simulink model "TO_ctr"  (R2017b)
settings: Solver=ode4  StartTime=0.0  StopTime=10  FixedStep=0.001  RelTol=1e-3
undefined symbols (not defined in the file or in its folder): MPC_alfa_tracking, MPC_TO_des_trq, sigbuilder_block
settings Model: Creator=Yutong Li  LastModifiedBy=Yutong Li

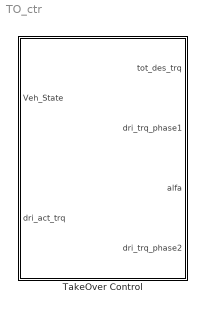
== system TO_ctr ==
  TakeOver Control : Subsystem

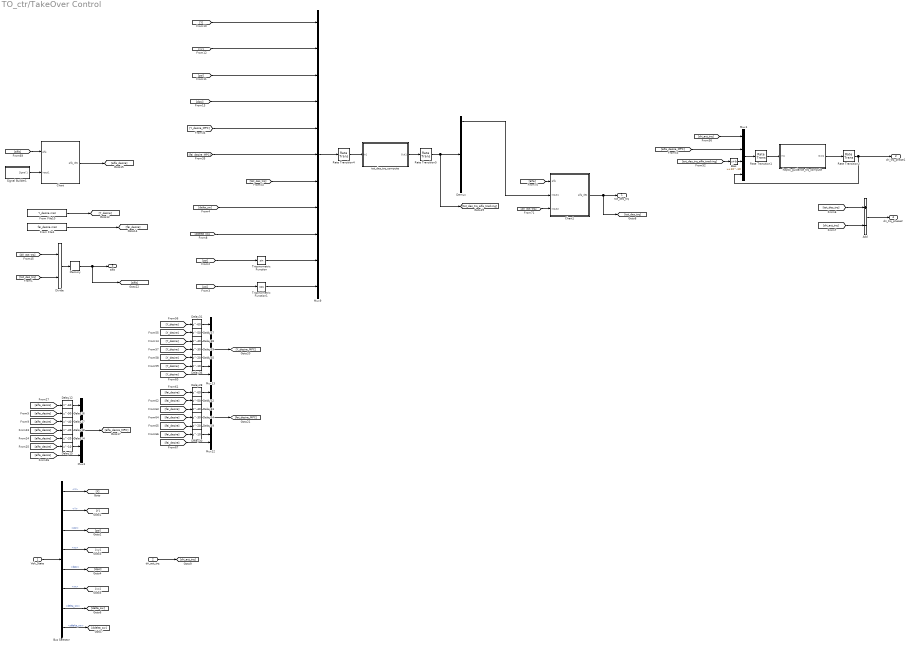
== system TO_ctr/TakeOver Control ==
  Veh_State : Inport
  dri_act_trq : Inport  Port=2
  Add : Sum  Inputs=+-
  Bias : Bias  Bias=10^-10
  Bus Selector : BusSelector  OutputSignals=X,Y,psi,vy,dpsi,vx,delta_sw,ddelta_sw
  Chart : Stateflow chart  TreatAsAtomicUnit=on
  Chart1 : Stateflow chart  TreatAsAtomicUnit=on
  Delay12 : Delay  DelayLength=60  InitialCondition=0
  Delay14 : Delay  DelayLength=20  InitialCondition=0
  Delay15 : Delay  DelayLength=10  InitialCondition=0
  Delay16 : Delay  DelayLength=50  InitialCondition=0
  Delay17 : Delay  DelayLength=40  InitialCondition=0
  Delay18 : Delay  DelayLength=30  InitialCondition=0
  Delay28 : Delay  DelayLength=60  InitialCondition=0
  Delay29 : Delay  DelayLength=20  InitialCondition=0
  Delay30 : Delay  DelayLength=10  InitialCondition=0
  Delay31 : Delay  DelayLength=60  InitialCondition=0
  Delay32 : Delay  DelayLength=50  InitialCondition=0
  Delay33 : Delay  DelayLength=40  InitialCondition=0
  Delay34 : Delay  DelayLength=30  InitialCondition=0
  Delay35 : Delay  DelayLength=20  InitialCondition=0
  Delay36 : Delay  DelayLength=10  InitialCondition=0
  Delay37 : Delay  DelayLength=50  InitialCondition=0
  Delay38 : Delay  DelayLength=40  InitialCondition=0
  Delay39 : Delay  DelayLength=30  InitialCondition=0
  Demux : Demux  Outputs=7
  Divide : Product  Inputs=*/
  From File1 : FromFile  FileName=fai_desire.mat
  From File10 : FromFile  FileName=Y_desire.mat
  Memory : Memory
  Mux1 : Mux
  Mux12 : Mux  Inputs=7
  Mux13 : Mux  Inputs=7
  Mux3 : Mux  Inputs=7
  Mux9 : Mux  Inputs=11
  Rate Transition1 : RateTransition  OutPortSampleTime=0.01
  Rate Transition2 : RateTransition
  Rate Transition4 : RateTransition  OutPortSampleTime=0.01
  Rate Transition5 : RateTransition
  Signal Builder1 : Subsystem  Tag=STV Subsys  LoadFcn=sigbuilder_block('load');  StartFcn=sigbuilder_block('start');  StopFcn=sigbuilder_block('stop');  ClipboardFcn=sigbuilder_block('clipboard');  mask(Sigbuilder block){tuvar=[0:10]}
      mask help: Simulink:masks:SigbuilderBlock_MD
      mask init:
      | if ~strcmp(get_param(bdroot(gcbh),'SimulationStatus'),'stopped') tuvar = sigbuilder_block('maskInit'); end
      settings: CopyFcn=sigbuilder_block('copy');  DeleteFcn=sigbuilder_block('delete');  ModelCloseFcn=sigbuilder_block('modelClose');  PreSaveFcn=sigbuilder_block('preSave');  PauseFcn=sigbuilder_block('pause');  ContinueFcn=sigbuilder_block('continue');  NameChangeFcn=sigbuilder_block('namechange');  OpenFcn=sigbuilder_block('open',[5.5 30 949 419 ]);  CloseFcn=sigbuilder_block('close');
      mask Display: plot(0, 0, 100, 100,[2, 2, 32, 32, 2], [68, 8, 8, 68, 68],[32, 2], [38, 38], [32, 19, 2],[53, 60, 44], [32, 17, 17, 2],[16, 16, 31, 31]);txt = getActiveGroup(gcbh);text(2, 100, txt,'verticalAlignment', 'top');
  Trigonometric Function : Trigonometry
  Trigonometric Function1 : Trigonometry  Operator=cos
  haptic_guidance_trq_compute : Subsystem  TreatAsAtomicUnit=on
  tot_des_trq_compute : Subsystem  TreatAsAtomicUnit=on
  tot_des_trq : Outport
  dri_trq_phase1 : Outport  Port=2
  alfa : Outport  Port=3
  dri_trq_phase2 : Outport  Port=4
  wires:
  Veh_State/1 -> Bus Selector/1
  Bus Selector/1 -> [X]  "<X>"
  Bus Selector/2 -> [Y]  "<Y>"
  Bus Selector/3 -> [psi]  "<psi>"
  Bus Selector/4 -> [vy]  "<vy>"
  Bus Selector/5 -> [dpsi]  "<dpsi>"
  Bus Selector/6 -> [vx]  "<vx>"
  [Y] -> Mux9/1
  [vy] -> Mux9/2
  [psi] -> Mux9/3
  [dpsi] -> Mux9/4
  From File10/1 -> [Y_desire]
  [alfa_desire] -> Delay14/1
  Delay16/1 -> Mux3/2
  [alfa_desire] -> Delay12/1
  [alfa_desire] -> Delay15/1
  [alfa_desire] -> Mux3/7
  [alfa_desire] -> Delay17/1
  Delay12/1 -> Mux3/1
  Delay14/1 -> Mux3/5
  Delay17/1 -> Mux3/3
  Delay18/1 -> Mux3/4
  [alfa_desire] -> Delay18/1
  [alfa_desire] -> Delay16/1
  Delay15/1 -> Mux3/6
  Mux3/1 -> [alfa_desire_MPC]
  [dri_act_trq] -> Divide/1
  [fai_desire_MPC] -> Mux9/6
  [Y_desire_MPC] -> Mux9/5
  Rate Transition4/1 -> tot_des_trq_compute/1(In1)
  tot_des_trq_compute/1(Out1) -> Rate Transition5/1
  Mux9/1 -> Rate Transition4/1
  Bus Selector/7 -> [delta_sw]  "<delta_sw>"
  Bus Selector/8 -> [ddelta_sw]  "<ddelta_sw>"
  [delta_sw] -> Mux9/8
  [ddelta_sw] -> Mux9/9
  [psi] -> Trigonometric Function/1
  Trigonometric Function/1 -> Mux9/10
  [psi] -> Trigonometric Function1/1
  Trigonometric Function1/1 -> Mux9/11
  Mux1/1 -> Rate Transition1/1
  Rate Transition1/1 -> haptic_guidance_trq_compute/1(In1)
  haptic_guidance_trq_compute/1(Out1) -> Rate Transition2/1
  Rate Transition2/1 -> dri_trq_phase1/1, Mux1/4
  dri_act_trq/1 -> [dri_act_trq]
  [tot_des_trq] -> Divide/2
  [dri_act_trq] -> Mux1/1
  [alfa_desire_MPC] -> Mux1/2
  [tot_des_trq_alfa_tracking] -> Bias/1
  Bias/1 -> Mux1/3
  Demux/1 -> Chart1/2(input1)
  [tot_des_trq] -> Mux9/7
  Rate Transition5/1 -> [tot_des_trq_alfa_tracking], Demux/1
  Mux12/1 -> [fai_desire_MPC]
  Delay36/1 -> Mux13/6
  Mux13/1 -> [Y_desire_MPC]
  [fai_desire] -> Delay29/1
  [fai_desire] -> Delay30/1
  [fai_desire] -> Delay33/1
  Delay29/1 -> Mux12/5
  Delay33/1 -> Mux12/3
  [fai_desire] -> Delay32/1
  Delay34/1 -> Mux12/4
  [Y_desire] -> Mux13/7
  [Y_desire] -> Delay38/1
  Delay37/1 -> Mux13/2
  [fai_desire] -> Delay28/1
  [Y_desire] -> Delay35/1
  Delay30/1 -> Mux12/6
  Delay38/1 -> Mux13/3
  [Y_desire] -> Delay37/1
  Delay32/1 -> Mux12/2
  [Y_desire] -> Delay39/1
  [fai_desire] -> Delay34/1
  [fai_desire] -> Mux12/7
  Delay31/1 -> Mux13/1
  Delay35/1 -> Mux13/5
  [Y_desire] -> Delay36/1
  Delay39/1 -> Mux13/4
  [Y_desire] -> Delay31/1
  Delay28/1 -> Mux12/1
  From File1/1 -> [fai_desire]
  Divide/1 -> Memory/1
  Signal Builder1/1(Signal 1) -> Chart/2(input1)
  Memory/1 -> [alfa], alfa/1
  Chart/1(alfa_des) -> [alfa_desire]
  [alfa] -> Chart/1(alfa)
  [alfa] -> Chart1/1(alfa)
  [dri_act_trq] -> Chart1/3(input2)
  Chart1/1(alfa_des) -> [tot_des_trq], tot_des_trq/1
  Add/1 -> dri_trq_phase2/1
  [tot_des_trq] -> Add/1
  [dri_act_trq] -> Add/2

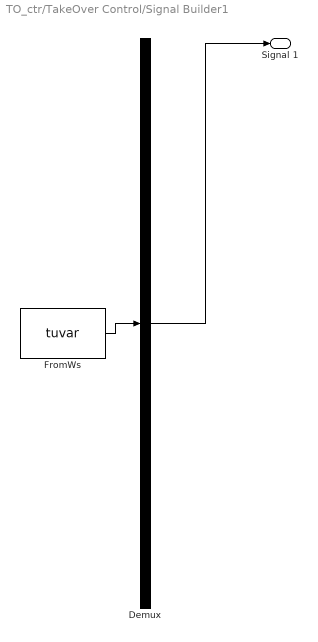
== system TO_ctr/TakeOver Control/Signal Builder1 ==
  Demux : Demux  Tag=STV Demux  Outputs=1
  FromWs : FromWorkspace  Tag=STV FromWs  VariableName=tuvar  SampleTime=0
      SigBuilderData=|
      | common.afterFinalStr = 'Extrapolate'
      | common.sampleTime = 0
      | dataSet.timeRange = [0 15]
      | dataSet.name = 'Group 1'
      | sbobj.Groups.Name = 'Group 1'
      | sbobj.Groups.Signals.Name = 'Signal 1'
      | sbobj.Groups.Signals.XData = [0 2 2 7.5 9.5 9.5 15]
      | sbobj.Groups.Signals.YData = [0 0 0.6 0.6 0.6 1 1]
      | sbobj.Groups.TimeRange = [0 15]
  Signal 1 : Outport  Tag=STV Outport
  wires:
  FromWs/1 -> Demux/1
  Demux/1 -> Signal 1/1

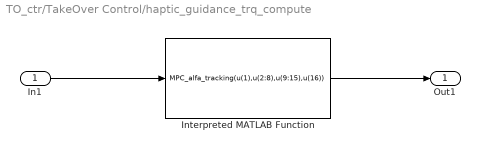
== system TO_ctr/TakeOver Control/haptic_guidance_trq_compute ==
  In1 : Inport
  Interpreted MATLAB Function : MATLABFcn  MATLABFcn=MPC_alfa_tracking(u(1),u(2:8),u(9:15),u(16))  OutputDimensions=1  SampleTime=0.01
  Out1 : Outport
  wires:
  Interpreted MATLAB Function/1 -> Out1/1
  In1/1 -> Interpreted MATLAB Function/1

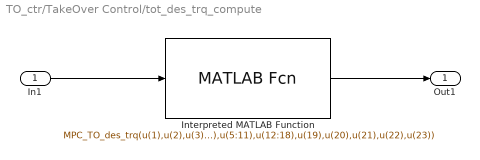
== system TO_ctr/TakeOver Control/tot_des_trq_compute ==
  In1 : Inport
  Interpreted MATLAB Function : MATLABFcn  MATLABFcn=MPC_TO_des_trq(u(1),u(2),u(3),u(4),u(5:11),u(12:18),u(19),u(20),u(21),u(22),u(23))  OutputDimensions=7  SampleTime=0.01
  Out1 : Outport
  wires:
  In1/1 -> Interpreted MATLAB Function/1
  Interpreted MATLAB Function/1 -> Out1/1

== stateflow chart TO_ctr/TakeOver Control/Chart ==
  state state_1
    during:
    alfa_des = input1;
  state state_2
    during:
    alfa_des = 0.9;
  state state_3
    during:
    alfa_des = 1;
  (default) -> state_1
  state_1 -> state_2 : [alfa>0.6]
  state_2 -> state_3 : [alfa>0.9]
  data: alfa input; input1 input; alfa_des output

== stateflow chart TO_ctr/TakeOver Control/Chart1 ==
  state state_1
    during:
    alfa_des = input1;
  state state_2
    during:
    alfa_des = input2;
  (default) -> state_1
  state_1 -> state_2 : [alfa>0.9]
  data: alfa input; input1 input; alfa_des output; input2 input
